simulink model "TV_2021"  (R2017b)
settings: Solver=VariableStepAuto  StartTime=0.0  StopTime=10.0  RelTol=1e-3
undefined symbols (not defined in the file): sigbuilder_block
libraries: simulink x6
(part 6 of 13)

== system TV_2021/Vehicle Dynamics Control 2018/VDC 2018 without Longitudinal/Driver // CarBehaviours ==
  Tq_FRin : Inport
  Tq_FLin : Inport  Port=2
  Tq_RRin : Inport  Port=3
  "Tq_RLin " : Inport  Port=4
  Bp : Inport  Port=5
  Ap : Inport  Port=6
  Reg_enable : Inport  Port=7
  Ap_Sat_up : Inport  Port=8
  Ap_Sat_down : Inport  Port=9
  Accelerating : Subsystem  TreatAsAtomicUnit=on
  "Accelerator behaviour " : MATLAB Function  TreatAsAtomicUnit=on
  Braking Conditions : If  NumInputs=3  IfExpression=u1>0 & u2<0.1 & u3==1  ElseIfExpressions=u1>0 & u2<0.1 & u3==0, u1<0.1 & u2<0.1
  Constant : Constant  Value=0
  Constant1 : Constant  Value=0
  Inertia Braking : Subsystem  TreatAsAtomicUnit=on
  Mech_Braking : Subsystem  TreatAsAtomicUnit=on
  Merge : Merge  Inputs=4
  Merge1 : Merge  Inputs=4
  Regenerative+Mech Braking : Subsystem  TreatAsAtomicUnit=on
  Terminator : Terminator
  Terminator1 : Terminator
  Tq_FRout : Outport
  "Tq_FLout " : Outport  Port=2
  Tq_RRout : Outport  Port=3
  Tq_RLout : Outport  Port=4
  out_Throttle : Outport  Port=5
  wires:
  Constant1/1 -> "Tq_FLout "/1
  Constant/1 -> Tq_FRout/1
  Tq_FLin/1 -> Terminator1/1
  Tq_FRin/1 -> Terminator/1
  Merge/1 -> Tq_RRout/1
  Merge1/1 -> Tq_RLout/1
  Bp/1 -> Braking Conditions/1
  Regenerative+Mech Braking/1("Tq_RR ") -> Merge/1
  Mech_Braking/1("Tq_RR ") -> Merge/2
  Inertia Braking/1("Tq_RR ") -> Merge/3
  Accelerating/1("Tq_RR ") -> Merge/4
  Regenerative+Mech Braking/2(Tq_RL) -> Merge1/1
  Mech_Braking/2(Tq_RL) -> Merge1/2
  Inertia Braking/2(Tq_RL) -> Merge1/3
  Accelerating/2(Tq_RL) -> Merge1/4
  Braking Conditions/1 -> Regenerative+Mech Braking/Action
  Braking Conditions/2 -> Mech_Braking/Action
  Braking Conditions/3 -> Inertia Braking/Action
  Braking Conditions/4 -> Accelerating/Action
  Tq_RRin/1 -> Accelerating/2(Tq_RR), Regenerative+Mech Braking/1(RegTq_RR)
  "Tq_RLin "/1 -> Accelerating/3("Tq_RL "), Regenerative+Mech Braking/2(RegTq_RL)
  Reg_enable/1 -> Braking Conditions/3
  Accelerating/3(Out_Throttle) -> out_Throttle/1
  "Accelerator behaviour "/1(throttle) -> Accelerating/1(Throttle), Braking Conditions/2
  Ap/1 -> "Accelerator behaviour "/1(Ap)
  Ap_Sat_up/1 -> "Accelerator behaviour "/2(Ap_Sat_up)
  Ap_Sat_down/1 -> "Accelerator behaviour "/3(Ap_Sat_down)

== system TV_2021/Vehicle Dynamics Control 2018/VDC 2018 without Longitudinal/In_Numbers ==
  C-Kamm_Factor : Inport
  Max Regen Torque [Nm] : Inport  Port=2
  Limit Power [kW] : Inport  Port=3
  Limit Temperature IGBT [ºC] : Inport  Port=4
  Limit Temperature Motor [ºC] : Inport  Port=5
  Reduction Power [0-1] : Inport  Port=6
  Reduction Temperature [0-1] : Inport  Port=7
  Steering Saturation (per site) [deg] : Inport  Port=8
  Ap_Sat_Down [-] : Inport  Port=9
  Ap_Sat_Up [-] : Inport  Port=10
  3% difference : Gain  Gain=0.97
  Effective Rolling Radius[inch] : Constant  Value=13
  Engine+Inverter Performance [-] : Constant  Value=0.8
  Maximum Torque per engine [Nm] : Constant  Value=140
  Maximum Transmission Torque Dynamic [Nm] : Constant  Value=140
  Maximum Transmission Torque Static [Nm] : Constant  Value=130
  Transmision Ratio[-] : Constant  Value=4
  inch to m : Gain  Gain=0.0254
  Steer_Sat [deg] : Outport
  Tq_Max [Nm] : Outport  Port=2
  Cornering Kamm_Factor [0-2] : Outport  Port=3
  Transmision_Ratio[-] : Outport  Port=4
  Effective Rolling Radius[m] : Outport  Port=5
  Ap_Sat_down[-] : Outport  Port=6
  Ap_Sat_up[-] : Outport  Port=7
  Engine+Inverter Performance[-] : Outport  Port=8
  Trans_max _static[Nm] : Outport  Port=9
  Trans_max_dynamic [Nm] : Outport  Port=10
  "Power limit [KW] " : Outport  Port=11
  Temperature limit IGBT [ºC] : Outport  Port=12
  Temperature limit Motor [ºC] : Outport  Port=13
  Reduction Power (0-1) : Outport  Port=14
  Reduction Temperature (0-1) : Outport  Port=15
  MaxRegTorque [Nm] : Outport  Port=16
  wires:
  Maximum Torque per engine [Nm]/1 -> Tq_Max [Nm]/1
  Transmision Ratio[-]/1 -> Transmision_Ratio[-]/1
  Effective Rolling Radius[inch]/1 -> inch to m/1
  Maximum Transmission Torque Static [Nm]/1 -> Trans_max _static[Nm]/1
  Maximum Transmission Torque Dynamic [Nm]/1 -> Trans_max_dynamic [Nm]/1
  inch to m/1 -> 3% difference/1
  3% difference/1 -> Effective Rolling Radius[m]/1
  Engine+Inverter Performance [-]/1 -> Engine+Inverter Performance[-]/1
  Max Regen Torque [Nm]/1 -> MaxRegTorque [Nm]/1
  Limit Power [kW]/1 -> "Power limit [KW] "/1
  Limit Temperature IGBT [ºC]/1 -> Temperature limit IGBT [ºC]/1
  Reduction Power [0-1]/1 -> Reduction Power (0-1)/1
  C-Kamm_Factor/1 -> Cornering Kamm_Factor [0-2]/1
  Steering Saturation (per site) [deg]/1 -> Steer_Sat [deg]/1
  Ap_Sat_Up [-]/1 -> Ap_Sat_up[-]/1
  Ap_Sat_Down [-]/1 -> Ap_Sat_down[-]/1
  Reduction Temperature [0-1]/1 -> Reduction Temperature (0-1)/1
  Limit Temperature Motor [ºC]/1 -> Temperature limit Motor [ºC]/1

== system TV_2021/Vehicle Dynamics Control 2018/VDC 2018 without Longitudinal/Kamm Circle Lateral ==
  "N_FR " : Inport
  N_FL : Inport  Port=2
  N_RR : Inport  Port=3
  N_RL : Inport  Port=4
  Fy : Inport  Port=5
  CK_Factor : Inport  Port=6
  Constant : Constant  Value=-1
  Constant1 : Constant  Value=-1
  Kamm_Circle LatD : MATLAB Function  TreatAsAtomicUnit=on
  MATLAB Function1 : MATLAB Function  TreatAsAtomicUnit=on
  MATLAB Function2 : MATLAB Function  TreatAsAtomicUnit=on
  Product : Product
  Product1 : Product
  Fx_FR : Outport
  Fx_FL : Outport  Port=2
  "Fx_RR " : Outport  Port=3
  "Fx_RL " : Outport  Port=4
  wires:
  N_FL/1 -> Fx_FL/1
  "N_FR "/1 -> Fx_FR/1
  N_RL/1 -> Kamm_Circle LatD/2(Fz_L)
  Fy/1 -> Kamm_Circle LatD/3(Fy)
  N_RR/1 -> Kamm_Circle LatD/1(Fz_R)
  Kamm_Circle LatD/1(Fx_R) -> Product/1
  Kamm_Circle LatD/2(Fx_L) -> Product1/1
  CK_Factor/1 -> Product/2, Product1/2
  Product1/1 -> MATLAB Function1/2(v)
  Product/1 -> MATLAB Function2/2(v)
  Constant1/1 -> MATLAB Function2/1(cte)
  MATLAB Function2/1(value) -> "Fx_RR "/1
  Constant/1 -> MATLAB Function1/1(cte)
  MATLAB Function1/1(value) -> "Fx_RL "/1

== system TV_2021/Vehicle Dynamics Control 2018/VDC 2018 without Longitudinal/Lateral Dynamics ==
  F_acc : Inport
  R_acc : Inport  Port=2
  FR_susp : Inport  Port=3
  FL_susp : Inport  Port=4
  RR_susp : Inport  Port=5
  RL_susp : Inport  Port=6
  Gas_pedal : Inport  Port=7
  Brake_pedal : Inport  Port=8
  Ellipse_acc : Inport  Port=9
  Constant1 : Constant  Value=0
  Constant2 : Constant  Value=0
  Demux : Demux  Outputs=3
  Demux1 : Demux  Outputs=3
  Fy per wheel : Gain  Gain=1/2
  Gravity : Gain  Gain=1/9.81
  Gravity1 : Gain  Gain=1/9.81
  Product : Product
  Sum : Sum  Inputs=++++
  Sum1 : Sum
  Sum2 : Sum  Inputs=+-
  Terminator{1..7} (7 alike) : Terminator
  N_FR : Outport
  "N_FL " : Outport  Port=2
  "N_RR " : Outport  Port=3
  N_RL : Outport  Port=4
  Fy_R : Outport  Port=5
  Mass [kg] (0,inf) : Outport  Port=6
  Handling [-] (-inf,inf) : Outport  Port=7
  wires:
  Constant2/1 -> "N_FL "/1
  Constant1/1 -> N_FR/1
  F_acc/1 -> Demux1/1
  Gas_pedal/1 -> Terminator4/1
  Brake_pedal/1 -> Terminator5/1
  Demux/2 -> Sum2/2, Product/1
  Demux/1 -> Terminator6/1
  Demux/3 -> Terminator3/1
  Product/1 -> Fy per wheel/1  "Fy per axe"
  Fy per wheel/1 -> Fy_R/1
  Gravity1/1 -> Product/2
  Sum/1 -> Gravity/1
  Sum1/1 -> Gravity1/1
  Gravity/1 -> Mass [kg] (0,inf)/1  "Mass [kg]"
  Demux1/1 -> Terminator1/1
  Demux1/3 -> Terminator2/1
  Demux1/2 -> Sum2/1
  Sum2/1 -> Handling [-] (-inf,inf)/1
  RL_susp/1 -> N_RL/1, Sum1/2, Sum/4
  RR_susp/1 -> Sum1/1, "N_RR "/1, Sum/3
  FL_susp/1 -> Sum/2
  FR_susp/1 -> Sum/1
  R_acc/1 -> Demux/1
  Ellipse_acc/1 -> Terminator7/1

== system TV_2021/Vehicle Dynamics Control 2018/VDC 2018 without Longitudinal/Optimization SKF & CKF ==
  RPM_INV1 : Inport
  RPM_INV2 : Inport  Port=2
  CKF_Initial : Inport  Port=3
  Cte_CKF : Inport  Port=4
  CKF_prev : DataStoreRead  DataStoreName=B
  Data Store Memory1 : DataStoreMemory  DataStoreName=B  ReadBeforeWriteMsg=warning  WriteAfterWriteMsg=warning  WriteAfterReadMsg=warning  ShowAdditionalParam=off
  Data Store Write1 : DataStoreWrite  DataStoreName=B
  Derivative : Derivative
  MATLAB Function : MATLAB Function  TreatAsAtomicUnit=on
  "Subsystem " : Subsystem
  CKF_act : Outport
  wires:
  CKF_prev/1 -> "Subsystem "/3("CKF_prev ")
  Derivative/1 -> "Subsystem "/1(Derivative)  "alpha"
  MATLAB Function/1(RPM) -> Derivative/1  "w (rad/s)"
  "Subsystem "/1(CKF_act) -> Data Store Write1/1, CKF_act/1  "CKF"
  Cte_CKF/1 -> "Subsystem "/4(Cte_CKF)
  CKF_Initial/1 -> "Subsystem "/2("CKF_Initial ")
  RPM_INV1/1 -> MATLAB Function/1(RPM_INV1)
  RPM_INV2/1 -> MATLAB Function/2(RPM_INV2)

== system TV_2021/Vehicle Dynamics Control 2018/VDC 2018 without Longitudinal/Sensor_DATA ==
  note: [ºC]
  note: [m/s2]
  note: [m/s2]
  note: [deg]
  note: [N]
  note: [N]
  note: [N]
  note: [N]
  note: [0-1]
  note: [0-1]
  note: [0 or 1]
  note: [0 - Inf]
  note: [rad/s]
  note: [rad/s]
  Steer_Ang : Inport
  "F_Acc " : Inport  Port=2
  R_Acc : Inport  Port=3
  FR_Susp : Inport  Port=4
  FL_Susp : Inport  Port=5
  RR_Susp : Inport  Port=6
  RL_Susp : Inport  Port=7
  Gas Pedal : Inport  Port=8
  Brake Pedal : Inport  Port=9
  Regenerative Enable : Inport  Port=10
  "Power " : Inport  Port=11
  TemperatureIGBT : Inport  Port=12
  TemperatureMotor : Inport  Port=13
  V_eRR : Inport  Port=14
  "V_eRL " : Inport  Port=15
  Ellipse_acc_ax_ay_az : Inport  Port=16
  Temp_Celdas : Inport  Port=17
  Lim_Temp_Celdas : Inport  Port=18
  Steer_ang : Outport
  F_acc : Outport  Port=2
  R_acc : Outport  Port=3
  FR_susp : Outport  Port=4
  FL_susp : Outport  Port=5
  RR_susp : Outport  Port=6
  RL_susp : Outport  Port=7
  Gas_Pedal : Outport  Port=8
  Brake_Pedal : Outport  Port=9
  Reg_Enable : Outport  Port=10
  Power : Outport  Port=11
  Temperature IGBT : Outport  Port=12
  Temperature Motor : Outport  Port=13
  "V_eRR " : Outport  Port=14
  V_eRL : Outport  Port=15
  Ellipse_acc : Outport  Port=16
  temp_celdas : Outport  Port=17  VectorParamsAs1DForOutWhenUnconnected=on
  Lim_temp_celdas : Outport  Port=18  VectorParamsAs1DForOutWhenUnconnected=on
  wires:
  RL_Susp/1 -> RL_susp/1
  RR_Susp/1 -> RR_susp/1
  FL_Susp/1 -> FL_susp/1
  FR_Susp/1 -> FR_susp/1
  Steer_Ang/1 -> Steer_ang/1
  R_Acc/1 -> R_acc/1
  "F_Acc "/1 -> F_acc/1
  Gas Pedal/1 -> Gas_Pedal/1
  Brake Pedal/1 -> Brake_Pedal/1
  Regenerative Enable/1 -> Reg_Enable/1
  "Power "/1 -> Power/1
  TemperatureIGBT/1 -> Temperature IGBT/1
  "V_eRL "/1 -> V_eRL/1
  V_eRR/1 -> "V_eRR "/1
  TemperatureMotor/1 -> Temperature Motor/1
  Ellipse_acc_ax_ay_az/1 -> Ellipse_acc/1
  Temp_Celdas/1 -> temp_celdas/1
  Lim_Temp_Celdas/1 -> Lim_temp_celdas/1

== system TV_2021/Vehicle Dynamics Control 2018/VDC 2018 without Longitudinal/Wheel_to_engine ==
  "Fx_FR " : Inport
  "Fx_FL " : Inport  Port=2
  "Fx_RR " : Inport  Port=3
  "Fx_RL " : Inport  Port=4
  Re : Inport  Port=5
  RT : Inport  Port=6
  Constant : Constant  Value=0
  Constant1 : Constant  Value=0
  Fx_to_engineTqRL : Subsystem
  Fx_to_engineTqRR : Subsystem
  MATLAB Function1 : MATLAB Function  TreatAsAtomicUnit=on
  MATLAB Function2 : MATLAB Function  TreatAsAtomicUnit=on
  Tq_FR : Outport
  Tq_FL : Outport  Port=2
  Tq_RR : Outport  Port=3
  Tq_RL : Outport  Port=4
  wires:
  Fx_to_engineTqRR/1(Tq) -> Tq_RR/1
  Fx_to_engineTqRL/1(Tq) -> Tq_RL/1
  "Fx_FR "/1 -> Tq_FR/1
  "Fx_FL "/1 -> Tq_FL/1
  Re/1 -> Fx_to_engineTqRR/2(Re), Fx_to_engineTqRL/2(Re)
  RT/1 -> Fx_to_engineTqRR/3(RT), Fx_to_engineTqRL/3(RT)
  "Fx_RR "/1 -> MATLAB Function2/2(v)
  "Fx_RL "/1 -> MATLAB Function1/2(v)
  MATLAB Function2/1(value) -> Fx_to_engineTqRR/1(Fx)
  Constant/1 -> MATLAB Function2/1(cte)
  Constant1/1 -> MATLAB Function1/1(cte)
  MATLAB Function1/1(value) -> Fx_to_engineTqRL/1(Fx)

== system TV_2021/If Action Subsystem1/Steering TV 2017 with TC/Constraints/Control de Potencia  ==
  Tq_RR : Inport
  Tq_RL : Inport  Port=2
  ReductionCte : Inport  Port=3
  Action Port : ActionPort
  Add : Sum  Inputs=+-
  Add1 : Sum  Inputs=+-
  Product : Product
  Product1 : Product
  Tq_RR_out : Outport
  Tq_RL_out : Outport  Port=2
  wires:
  Tq_RR/1 -> Product/1, Add/1
  Tq_RL/1 -> Product1/1, Add1/1
  ReductionCte/1 -> Product/2, Product1/2
  Product1/1 -> Add1/2
  Product/1 -> Add/2
  Add1/1 -> Tq_RL_out/1
  Add/1 -> Tq_RR_out/1

== system TV_2021/If Action Subsystem1/Steering TV 2017 with TC/Constraints/Control de Temperatura ==
  Tq_RR : Inport
  Tq_RL : Inport  Port=2
  ReductionCte : Inport  Port=3
  Action Port : ActionPort
  Add : Sum  Inputs=+-
  Add1 : Sum  Inputs=+-
  Product : Product
  Product1 : Product
  Tq_RR_out : Outport
  Tq_RL_out : Outport  Port=2
  wires:
  Add/1 -> Tq_RR_out/1
  Add1/1 -> Tq_RL_out/1
  Product/1 -> Add/2
  Product1/1 -> Add1/2
  ReductionCte/1 -> Product1/2, Product/2
  Tq_RL/1 -> Add1/1, Product1/1
  Tq_RR/1 -> Add/1, Product/1

== system TV_2021/If Action Subsystem1/Steering TV 2017 with TC/Constraints/else ==
  Tq_RR : Inport
  Tq_RL : Inport  Port=2
  Action Port : ActionPort
  Tq_RR_out : Outport
  Tq_RL_out : Outport  Port=2
  wires:
  Tq_RR/1 -> Tq_RR_out/1
  Tq_RL/1 -> Tq_RL_out/1

== system TV_2021/If Action Subsystem1/Steering TV 2017 with TC/Optimization SKF & CKF/Subsystem  ==
  Steer_An : Inport
  Derivative : Inport  Port=2
  SKF_Initial : Inport  Port=3
  SKF_prev : Inport  Port=4
  "CKF_Initial " : Inport  Port=5
  "CKF_prev " : Inport  Port=6
  Cte_SKF : Inport  Port=7
  Cte_CKF : Inport  Port=8
  CKF : Subsystem
  MATLAB Function1 : MATLAB Function  TreatAsAtomicUnit=on
  SKF : Subsystem
  SKF or CKF : If  IfExpression=-10 < u1 & u1 < 10
  Steering Wheel Maximum Angle : Constant  Value=100
  "SKF_act " : Outport
  CKF_act : Outport  Port=2
  wires:
  MATLAB Function1/1(value) -> SKF or CKF/1
  Steering Wheel Maximum Angle/1 -> MATLAB Function1/1(cte)
  Steer_An/1 -> MATLAB Function1/2(v)
  SKF/1(SKF_act) -> "SKF_act "/1
  CKF/1("CKF_act ") -> CKF_act/1
  SKF or CKF/1 -> SKF/Action
  SKF or CKF/2 -> CKF/Action
  "CKF_prev "/1 -> CKF/3("CKF_prev ")
  Derivative/1 -> CKF/1(Derivative), SKF/1(Derivative)
  SKF_Initial/1 -> SKF/2("SKF_Initial ")
  SKF_prev/1 -> SKF/3(SKF_prev)
  "CKF_Initial "/1 -> CKF/2(CKF_Initial)
  Cte_SKF/1 -> SKF/4(Cte_SKF)
  Cte_CKF/1 -> CKF/4(Cte_CKF)

== system TV_2021/If Action Subsystem1/VDC 2018 Complete/Constraints/Acelerating and braking without Regenerative ==
  Tq_max : Inport
  V_eRR : Inport  Port=2
  V_eRL : Inport  Port=3
  Trans_max_dynamic : Inport  Port=4
  Trans_max_static : Inport  Port=5
  Power_limit : Inport  Port=6
  Power : Inport  Port=7
  Temperature_limit_IGBT : Inport  Port=8
  TemperatureIGBT : Inport  Port=9
  TemperatureI_limit_Motor : Inport  Port=10
  TemperatureMotor : Inport  Port=11
  ReductionCte_Power : Inport  Port=12
  ReductionCte_Temperature : Inport  Port=13
  Tq_FR : Inport  Port=14
  Tq_FL : Inport  Port=15
  Tq_RR : Inport  Port=16
  Tq_RL : Inport  Port=17
  Tq_diff : Inport  Port=18
  Action Port : ActionPort
  "Control de Potencia " : Subsystem  TreatAsAtomicUnit=on
  Control de Temperatura : Subsystem  TreatAsAtomicUnit=on
  Gain : Gain  Gain=3.141592/30
  If : If  NumInputs=6  IfExpression=u4 >= u3 | u6 >= u5  ElseIfExpressions=u2 >= u1
  If Action 1 : Subsystem  TreatAsAtomicUnit=on
  If Action 2 : Subsystem  TreatAsAtomicUnit=on
  If1 : If  NumInputs=3  IfExpression=u1 > u3 & u2 > u3
  Merge{,1,3..4} (4 alike) : Merge  Inputs=3
  Merge2 : Merge
  Momentum Z scaled : Subsystem
  Terminator : Terminator
  Terminator1 : Terminator
  else : Subsystem  TreatAsAtomicUnit=on
  minimum value : MATLAB Function  TreatAsAtomicUnit=on
  minimum value1 : MATLAB Function  TreatAsAtomicUnit=on
  rpm : Constant  Value=200
  TQ_RR : Outport
  TQ_RL : Outport  Port=2
  Flag_Temperature : Outport  Port=3
  Flag_Power : Outport  Port=4
  wires:
  If1/1 -> If Action 1/Action
  If Action 1/1(Trans_limit) -> Merge2/1
  Merge2/1 -> minimum value/1(a), minimum value1/1(a)
  Trans_max_dynamic/1 -> If Action 1/1(Trans_max_dynamic)
  If Action 2/1(Trans_limit) -> Merge2/2
  V_eRR/1 -> If1/1
  V_eRL/1 -> If1/2
  If1/2 -> If Action 2/Action
  Trans_max_static/1 -> If Action 2/1("Trans_max_static ")
  Tq_max/1 -> minimum value1/2(b), minimum value/2(b)
  rpm/1 -> Gain/1
  Gain/1 -> If1/3  "approx 20.95"
  Tq_FR/1 -> Terminator/1
  Tq_FL/1 -> Terminator1/1
  TemperatureIGBT/1 -> If/4
  ReductionCte_Power/1 -> "Control de Potencia "/3(ReductionCte)
  If/3 -> else/Action
  Power_limit/1 -> If/1
  Power/1 -> If/2
  Temperature_limit_IGBT/1 -> If/3
  minimum value/1(min) -> Control de Temperatura/1(Tq_RR), "Control de Potencia "/1(Tq_RR), else/1(Tq_RR)
  minimum value1/1(min) -> Control de Temperatura/2(Tq_RL), "Control de Potencia "/2(Tq_RL), else/2(Tq_RL)
  ReductionCte_Temperature/1 -> Control de Temperatura/3(ReductionCte)
  "Control de Potencia "/1(Tq_RR_out) -> Merge/1
  Control de Temperatura/1(Tq_RR_out) -> Merge/2
  else/1(Tq_RR_out) -> Merge/3
  "Control de Potencia "/2(Tq_RL_out) -> Merge1/1
  Control de Temperatura/2(Tq_RL_out) -> Merge1/2
  else/2(Tq_RL_out) -> Merge1/3
  If/1 -> Control de Temperatura/Action
  If/2 -> "Control de Potencia "/Action
  Tq_RR/1 -> [tq_RR_wc], minimum value/3(c)
  Tq_RL/1 -> [tq_RL_wc], minimum value1/3(c)
  Merge/1 -> Momentum Z scaled/1(Tq_RR_Lim)
  Merge1/1 -> Momentum Z scaled/2(Tq_RL_Lim)
  [tq_RR_wc] -> Momentum Z scaled/3(Tq_RR_wc)
  [tq_RL_wc] -> Momentum Z scaled/4(Tq_RL_wc)
  TemperatureI_limit_Motor/1 -> If/5
  TemperatureMotor/1 -> If/6
  Merge3/1 -> Flag_Temperature/1
  Merge4/1 -> Flag_Power/1
  Control de Temperatura/3(Flag_Temperature) -> Merge3/1
  Control de Temperatura/4(Flag_Power) -> Merge4/1
  "Control de Potencia "/3(Flag_Temperature) -> Merge3/2
  "Control de Potencia "/4(Flag_Power) -> Merge4/2
  else/3(Flag_Temperature) -> Merge3/3
  else/4(Flag_Power) -> Merge4/3
  Momentum Z scaled/1(TQ_RR) -> TQ_RR/1
  Momentum Z scaled/2(TQ_RL) -> TQ_RL/1
  Tq_diff/1 -> Momentum Z scaled/5(Tq_diff)

== system TV_2021/If Action Subsystem1/VDC 2018 Complete/Constraints/Braking with Regenerative ==
  MaxRegTorque : Inport
  Tq_RR_wc : Inport  Port=2
  Tq_RL_wc : Inport  Port=3
  Action Port : ActionPort
  Gain : Gain  Gain=-1
  Gain1 : Gain  Gain=-1
  MATLAB Function : MATLAB Function  TreatAsAtomicUnit=on
  TQ_RR : Outport
  TQ_RL : Outport  Port=2
  wires:
  MATLAB Function/2(RegTq_RL) -> Gain1/1
  MATLAB Function/1(RegTq_RR) -> Gain/1
  Tq_RR_wc/1 -> MATLAB Function/2(Tq_RR)
  Tq_RL_wc/1 -> MATLAB Function/3(Tq_RL)
  MaxRegTorque/1 -> MATLAB Function/1(MaxRegenTq)
  Gain1/1 -> TQ_RL/1
  Gain/1 -> TQ_RR/1

== system TV_2021/If Action Subsystem1/VDC 2018 Complete/Driver // CarBehaviours/Accelerating ==
  Throttle : Inport
  Tq_RR : Inport  Port=2
  "Tq_RL " : Inport  Port=3
  Action Port : ActionPort
  Product : Product
  Product1 : Product
  "Tq_RR " : Outport
  Tq_RL : Outport  Port=2
  Out_Throttle : Outport  Port=3
  wires:
  Product1/1 -> "Tq_RR "/1
  Product/1 -> Tq_RL/1
  Throttle/1 -> Out_Throttle/1, Product/1, Product1/1
  Tq_RR/1 -> Product1/2
  "Tq_RL "/1 -> Product/2

== system TV_2021/If Action Subsystem1/VDC 2018 Complete/Driver // CarBehaviours/Inertia Braking ==
  Action Port : ActionPort
  Constant : Constant  Value=0
  Constant1 : Constant  Value=0
  "Tq_RR " : Outport
  Tq_RL : Outport  Port=2
  wires:
  Constant1/1 -> Tq_RL/1
  Constant/1 -> "Tq_RR "/1

== system TV_2021/If Action Subsystem1/VDC 2018 Complete/Driver // CarBehaviours/Mech_Braking ==
  Action Port : ActionPort
  Constant : Constant  Value=0
  Constant1 : Constant  Value=0
  "Tq_RR " : Outport
  Tq_RL : Outport  Port=2
  wires:
  Constant1/1 -> Tq_RL/1
  Constant/1 -> "Tq_RR "/1

== system TV_2021/If Action Subsystem1/VDC 2018 Complete/Driver // CarBehaviours/Regenerative+Mech Braking ==
  RegTq_RR : Inport
  RegTq_RL : Inport  Port=2
  Action Port : ActionPort
  "Tq_RR " : Outport
  Tq_RL : Outport  Port=2
  wires:
  RegTq_RR/1 -> "Tq_RR "/1
  RegTq_RL/1 -> Tq_RL/1

== system TV_2021/If Action Subsystem1/VDC 2018 Complete/Lateral Dynamics/Kamm_Circle ==
  Fz_R : Inport
  Fz_L : Inport  Port=2
  Fy : Inport  Port=3
  CK_Factor : Inport  Port=4
  Kamm_Circle LatD : MATLAB Function  TreatAsAtomicUnit=on
  Product1 : Product
  Product2 : Product
  Fx_R : Outport
  Fx_L : Outport  Port=2
  Fy_R [N] (0,inf) : Outport  Port=3
  wires:
  Product1/1 -> Fx_R/1
  CK_Factor/1 -> Product1/2, Product2/2
  Product2/1 -> Fx_L/1
  Kamm_Circle LatD/2(Fx_L) -> Product2/1
  Kamm_Circle LatD/1(Fx_R) -> Product1/1
  Fy/1 -> Kamm_Circle LatD/3(Fy)
  Fz_R/1 -> Kamm_Circle LatD/1(Fz_R)
  Fz_L/1 -> Kamm_Circle LatD/2(Fz_L)
  Kamm_Circle LatD/3(Fy_R) -> Fy_R [N] (0,inf)/1

== system TV_2021/If Action Subsystem1/VDC 2018 Complete/Lateral Dynamics/Racecar Model Constants ==
  Wheelbase [m] : Inport
  C. Stiffness [N/rad] : Inport  Port=2
  Steering_Ratio [-] : Inport  Port=3
  L (m) : Outport
  C (N/rad) : Outport  Port=2
  st_ratio (-) : Outport  Port=3
  wires:
  Wheelbase [m]/1 -> L (m)/1
  Steering_Ratio [-]/1 -> st_ratio (-)/1
  C. Stiffness [N/rad]/1 -> C (N/rad)/1

== system TV_2021/If Action Subsystem1/VDC 2018 Complete/Longitudinal Dynamics/Kamm_Circle ==
  Fz_R : Inport
  Fz_L : Inport  Port=2
  Fy : Inport  Port=3
  SK_Factor : Inport  Port=4
  Kamm_Circle LatD : MATLAB Function  TreatAsAtomicUnit=on
  Product : Product
  Product1 : Product
  Fx_R : Outport
  Fx_L : Outport  Port=2
  wires:
  Kamm_Circle LatD/1(Fx_R) -> Product/1
  Kamm_Circle LatD/2(Fx_L) -> Product1/1
  Fz_L/1 -> Kamm_Circle LatD/2(Fz_L)
  Fy/1 -> Kamm_Circle LatD/3(Fy)
  SK_Factor/1 -> Product/2, Product1/2
  Product/1 -> Fx_R/1
  Product1/1 -> Fx_L/1
  Fz_R/1 -> Kamm_Circle LatD/1(Fz_R)

== system TV_2021/If Action Subsystem1/VDC 2018 Complete/Optimization SKF & CKF/Subsystem  ==
  Steer_An : Inport
  Derivative : Inport  Port=2
  SKF_Initial : Inport  Port=3
  SKF_prev : Inport  Port=4
  "CKF_Initial " : Inport  Port=5
  "CKF_prev " : Inport  Port=6
  Cte_SKF : Inport  Port=7
  Cte_CKF : Inport  Port=8
  CKF : Subsystem
  MATLAB Function1 : MATLAB Function  TreatAsAtomicUnit=on
  SKF : Subsystem
  SKF or CKF : If  IfExpression=-10 < u1 & u1 < 10
  Steering Wheel Maximum Angle : Constant  Value=100
  "SKF_act " : Outport
  CKF_act : Outport  Port=2
  wires:
  MATLAB Function1/1(value) -> SKF or CKF/1
  Steering Wheel Maximum Angle/1 -> MATLAB Function1/1(cte)
  Steer_An/1 -> MATLAB Function1/2(v)
  SKF/1(SKF_act) -> "SKF_act "/1
  CKF/1("CKF_act ") -> CKF_act/1
  SKF or CKF/1 -> SKF/Action
  SKF or CKF/2 -> CKF/Action
  "CKF_prev "/1 -> CKF/3("CKF_prev ")
  Derivative/1 -> CKF/1(Derivative), SKF/1(Derivative)
  SKF_Initial/1 -> SKF/2("SKF_Initial ")
  SKF_prev/1 -> SKF/3(SKF_prev)
  "CKF_Initial "/1 -> CKF/2(CKF_Initial)
  Cte_SKF/1 -> SKF/4(Cte_SKF)
  Cte_CKF/1 -> CKF/4(Cte_CKF)

== system TV_2021/If Action Subsystem1/VDC 2018 Complete/Wheel_to_engine/Fx_to_engineTqRL ==
  Fx : Inport
  Re : Inport  Port=2
  RT : Inport  Port=3
  Divide : Product  Inputs=*/
  Product : Product
  Tq : Outport
  wires:
  Divide/1 -> Tq/1
  Product/1 -> Divide/1
  RT/1 -> Divide/2
  Fx/1 -> Product/1
  Re/1 -> Product/2

== system TV_2021/If Action Subsystem1/VDC 2018 Complete/Wheel_to_engine/Fx_to_engineTqRR ==
  Fx : Inport
  Re : Inport  Port=2
  RT : Inport  Port=3
  Divide : Product  Inputs=*/
  Product : Product
  Tq : Outport
  wires:
  Divide/1 -> Tq/1
  Product/1 -> Divide/1
  RT/1 -> Divide/2
  Fx/1 -> Product/1
  Re/1 -> Product/2

== system TV_2021/If Action Subsystem1/VDC 2018 without Longitudinal/Constraints/Acelerating and braking without Regenerative ==
  Tq_max : Inport
  V_eRR : Inport  Port=2
  V_eRL : Inport  Port=3
  Trans_max_dynamic : Inport  Port=4
  Trans_max_static : Inport  Port=5
  Power_limit : Inport  Port=6
  Power : Inport  Port=7
  Temperature_limit_IGBT : Inport  Port=8
  TemperatureIGBT : Inport  Port=9
  TemperatureI_limit_Motor : Inport  Port=10
  TemperatureMotor : Inport  Port=11
  ReductionCte_Power : Inport  Port=12
  ReductionCte_Temperature : Inport  Port=13
  Tq_FR : Inport  Port=14
  Tq_FL : Inport  Port=15
  Tq_RR : Inport  Port=16
  Tq_RL : Inport  Port=17
  Action Port : ActionPort
  "Control de Potencia " : Subsystem  TreatAsAtomicUnit=on
  Control de Temperatura : Subsystem  TreatAsAtomicUnit=on
  Gain : Gain  Gain=3.141592/30
  If : If  NumInputs=6  IfExpression=u4 >= u3 | u6 >= u5  ElseIfExpressions=u2 >= u1
  If Action 1 : Subsystem  TreatAsAtomicUnit=on
  If Action 2 : Subsystem  TreatAsAtomicUnit=on
  If1 : If  NumInputs=3  IfExpression=u1 > u3 & u2 > u3
  Merge : Merge  Inputs=3
  Merge1 : Merge  Inputs=3
  Merge2 : Merge
  Momentum Z scaled : Subsystem
  Terminator : Terminator
  Terminator1 : Terminator
  else : Subsystem  TreatAsAtomicUnit=on
  minimum value : MATLAB Function  TreatAsAtomicUnit=on
  minimum value1 : MATLAB Function  TreatAsAtomicUnit=on
  rpm : Constant  Value=200
  TQ_RR : Outport
  TQ_RL : Outport  Port=2
  wires:
  If1/1 -> If Action 1/Action
  If Action 1/1(Trans_limit) -> Merge2/1
  Merge2/1 -> minimum value/1(a), minimum value1/1(a)
  Trans_max_dynamic/1 -> If Action 1/1(Trans_max_dynamic)
  If Action 2/1(Trans_limit) -> Merge2/2
  V_eRR/1 -> If1/1
  V_eRL/1 -> If1/2
  If1/2 -> If Action 2/Action
  Trans_max_static/1 -> If Action 2/1("Trans_max_static ")
  Tq_max/1 -> minimum value1/2(b), minimum value/2(b)
  rpm/1 -> Gain/1
  Gain/1 -> If1/3  "approx 20.95"
  Tq_FR/1 -> Terminator/1
  Tq_FL/1 -> Terminator1/1
  TemperatureIGBT/1 -> If/4
  ReductionCte_Power/1 -> "Control de Potencia "/3(ReductionCte)
  If/3 -> else/Action
  Power_limit/1 -> If/1
  Power/1 -> If/2
  Temperature_limit_IGBT/1 -> If/3
  minimum value/1(min) -> Control de Temperatura/1(Tq_RR), "Control de Potencia "/1(Tq_RR), else/1(Tq_RR)
  minimum value1/1(min) -> Control de Temperatura/2(Tq_RL), "Control de Potencia "/2(Tq_RL), else/2(Tq_RL)
  ReductionCte_Temperature/1 -> Control de Temperatura/3(ReductionCte)
  "Control de Potencia "/1(Tq_RR_out) -> Merge/1
  Control de Temperatura/1(Tq_RR_out) -> Merge/2
  else/1(Tq_RR_out) -> Merge/3
  "Control de Potencia "/2(Tq_RL_out) -> Merge1/1
  Control de Temperatura/2(Tq_RL_out) -> Merge1/2
  else/2(Tq_RL_out) -> Merge1/3
  If/1 -> Control de Temperatura/Action
  If/2 -> "Control de Potencia "/Action
  Tq_RR/1 -> [tq_RR_wc], minimum value/3(c)
  Tq_RL/1 -> [tq_RL_wc], minimum value1/3(c)
  Merge/1 -> Momentum Z scaled/1(Tq_RR_Lim)
  Merge1/1 -> Momentum Z scaled/2(Tq_RL_Lim)
  [tq_RR_wc] -> Momentum Z scaled/3(Tq_RR_wc)
  [tq_RL_wc] -> Momentum Z scaled/4(Tq_RL_wc)
  TemperatureI_limit_Motor/1 -> If/5
  TemperatureMotor/1 -> If/6
  Momentum Z scaled/1(TQ_RR) -> TQ_RR/1
  Momentum Z scaled/2(TQ_RL) -> TQ_RL/1

== system TV_2021/If Action Subsystem1/VDC 2018 without Longitudinal/Constraints/Braking with Regenerative ==
  MaxRegTorque : Inport
  Tq_RR_wc : Inport  Port=2
  Tq_RL_wc : Inport  Port=3
  Action Port : ActionPort
  Gain : Gain  Gain=-1
  Gain1 : Gain  Gain=-1
  MATLAB Function : MATLAB Function  TreatAsAtomicUnit=on
  TQ_RR : Outport
  TQ_RL : Outport  Port=2
  wires:
  MATLAB Function/2(RegTq_RL) -> Gain1/1
  MATLAB Function/1(RegTq_RR) -> Gain/1
  Tq_RR_wc/1 -> MATLAB Function/2(Tq_RR)
  Tq_RL_wc/1 -> MATLAB Function/3(Tq_RL)
  MaxRegTorque/1 -> MATLAB Function/1(MaxRegenTq)
  Gain1/1 -> TQ_RL/1
  Gain/1 -> TQ_RR/1

== system TV_2021/If Action Subsystem1/VDC 2018 without Longitudinal/Driver // CarBehaviours/Accelerating ==
  Ap : Inport
  "Ap_Sat_up " : Inport  Port=2
  Ap_Sat_down : Inport  Port=3
  Tq_RR : Inport  Port=4
  "Tq_RL " : Inport  Port=5
  Action Port : ActionPort
  "Accelerator behaviour " : MATLAB Function  TreatAsAtomicUnit=on
  Product : Product
  Product1 : Product
  "Tq_RR " : Outport
  Tq_RL : Outport  Port=2
  Out_Throttle : Outport  Port=3
  wires:
  Ap/1 -> "Accelerator behaviour "/1(Ap)
  "Ap_Sat_up "/1 -> "Accelerator behaviour "/2(Ap_Sat_up)
  Ap_Sat_down/1 -> "Accelerator behaviour "/3(Ap_Sat_down)
  Product1/1 -> "Tq_RR "/1
  Product/1 -> Tq_RL/1
  "Accelerator behaviour "/1(throttle) -> Out_Throttle/1, Product/1, Product1/1
  Tq_RR/1 -> Product1/2
  "Tq_RL "/1 -> Product/2

== system TV_2021/If Action Subsystem1/VDC 2018 without Longitudinal/Driver // CarBehaviours/Inertia Braking ==
  Action Port : ActionPort
  Constant : Constant  Value=0
  Constant1 : Constant  Value=0
  "Tq_RR " : Outport
  Tq_RL : Outport  Port=2
  wires:
  Constant1/1 -> Tq_RL/1
  Constant/1 -> "Tq_RR "/1

== system TV_2021/If Action Subsystem1/VDC 2018 without Longitudinal/Driver // CarBehaviours/Mech_Braking ==
  Action Port : ActionPort
  Constant : Constant  Value=0
  Constant1 : Constant  Value=0
  "Tq_RR " : Outport
  Tq_RL : Outport  Port=2
  wires:
  Constant1/1 -> Tq_RL/1
  Constant/1 -> "Tq_RR "/1

== system TV_2021/If Action Subsystem1/VDC 2018 without Longitudinal/Driver // CarBehaviours/Regenerative+Mech Braking ==
  RegTq_RR : Inport
  RegTq_RL : Inport  Port=2
  Action Port : ActionPort
  "Tq_RR " : Outport
  Tq_RL : Outport  Port=2
  wires:
  RegTq_RL/1 -> Tq_RL/1
  RegTq_RR/1 -> "Tq_RR "/1

== system TV_2021/If Action Subsystem1/VDC 2018 without Longitudinal/Optimization SKF & CKF/Subsystem  ==
  Derivative : Inport
  "CKF_Initial " : Inport  Port=2
  "CKF_prev " : Inport  Port=3
  Cte_CKF : Inport  Port=4
  CKF : Subsystem
  CKF_act : Outport
  wires:
  CKF/1("CKF_act ") -> CKF_act/1
  "CKF_prev "/1 -> CKF/3("CKF_prev ")
  Derivative/1 -> CKF/1(Derivative)
  "CKF_Initial "/1 -> CKF/2(CKF_Initial)
  Cte_CKF/1 -> CKF/4(Cte_CKF)

== system TV_2021/If Action Subsystem1/VDC 2018 without Longitudinal/Wheel_to_engine/Fx_to_engineTqRL ==
  Fx : Inport
  Re : Inport  Port=2
  RT : Inport  Port=3
  Divide : Product  Inputs=*/
  Product : Product
  Tq : Outport
  wires:
  Divide/1 -> Tq/1
  Product/1 -> Divide/1
  RT/1 -> Divide/2
  Fx/1 -> Product/1
  Re/1 -> Product/2

== system TV_2021/If Action Subsystem1/VDC 2018 without Longitudinal/Wheel_to_engine/Fx_to_engineTqRR ==
  Fx : Inport
  Re : Inport  Port=2
  RT : Inport  Port=3
  Divide : Product  Inputs=*/
  Product : Product
  Tq : Outport
  wires:
  Divide/1 -> Tq/1
  Product/1 -> Divide/1
  RT/1 -> Divide/2
  Fx/1 -> Product/1
  Re/1 -> Product/2

== system TV_2021/Vehicle Dynamics Control 1/Steering TV 2017 with TC/Constraints/Control de Potencia  ==
  Tq_RR : Inport
  Tq_RL : Inport  Port=2
  ReductionCte : Inport  Port=3
  Action Port : ActionPort
  Add : Sum  Inputs=+-
  Add1 : Sum  Inputs=+-
  Product : Product
  Product1 : Product
  Tq_RR_out : Outport
  Tq_RL_out : Outport  Port=2
  wires:
  Add/1 -> Tq_RR_out/1
  Add1/1 -> Tq_RL_out/1
  Product/1 -> Add/2
  Product1/1 -> Add1/2
  ReductionCte/1 -> Product1/2, Product/2
  Tq_RL/1 -> Add1/1, Product1/1
  Tq_RR/1 -> Add/1, Product/1

== system TV_2021/Vehicle Dynamics Control 1/Steering TV 2017 with TC/Constraints/Control de Temperatura ==
  Tq_RR : Inport
  Tq_RL : Inport  Port=2
  ReductionCte : Inport  Port=3
  Action Port : ActionPort
  Add : Sum  Inputs=+-
  Add1 : Sum  Inputs=+-
  Product : Product
  Product1 : Product
  Tq_RR_out : Outport
  Tq_RL_out : Outport  Port=2
  wires:
  Add/1 -> Tq_RR_out/1
  ReductionCte/1 -> Product/2, Product1/2
  Tq_RL/1 -> Product1/1, Add1/1
  Tq_RR/1 -> Product/1, Add/1
  Add1/1 -> Tq_RL_out/1
  Product1/1 -> Add1/2
  Product/1 -> Add/2

== system TV_2021/Vehicle Dynamics Control 1/Steering TV 2017 with TC/Constraints/current_limitation1 ==
  note: % de la corriente total que te dejo usar
  max_cell_temp : Inport
  actual_current : Inport  Port=2
  initial_limitation : Inport  Port=3
  max_discharge_current : Inport  Port=4
  max_regen_current : Inport  Port=5
  Product1 : Product
  constants_saturator : Subsystem
  temperature_rise_limitator : Subsystem
  max_discharge (-) : Outport  VectorParamsAs1DForOutWhenUnconnected=on
  max_regen (+) : Outport  Port=2  VectorParamsAs1DForOutWhenUnconnected=on
  fans_control : Outport  Port=3  VectorParamsAs1DForOutWhenUnconnected=on
  wires:
  temperature_rise_limitator/1(allowed_current) -> Product1/1, fans_control/1
  max_regen_current/1 -> constants_saturator/3(max_regen_current)
  max_discharge_current/1 -> constants_saturator/2(max_discharge_current)
  initial_limitation/1 -> temperature_rise_limitator/2(initial_limitation)
  constants_saturator/2(limited_regen_actual) -> max_regen (+)/1
  constants_saturator/1(limited_discharge_actual) -> max_discharge (-)/1
  Product1/1 -> constants_saturator/1(allowed_current [%])
  max_cell_temp/1 -> temperature_rise_limitator/1(max_cell_temp)
  actual_current/1 -> Product1/2

== system TV_2021/Vehicle Dynamics Control 1/Steering TV 2017 with TC/Constraints/else ==
  Tq_RR : Inport
  Tq_RL : Inport  Port=2
  Action Port : ActionPort
  Tq_RR_out : Outport
  Tq_RL_out : Outport  Port=2
  wires:
  Tq_RL/1 -> Tq_RL_out/1
  Tq_RR/1 -> Tq_RR_out/1

== system TV_2021/Vehicle Dynamics Control 1/Steering TV 2017 with TC/Optimization SKF & CKF/Subsystem  ==
  Steer_An : Inport
  Derivative : Inport  Port=2
  SKF_Initial : Inport  Port=3
  SKF_prev : Inport  Port=4
  "CKF_Initial " : Inport  Port=5
  "CKF_prev " : Inport  Port=6
  Cte_SKF : Inport  Port=7
  Cte_CKF : Inport  Port=8
  CKF : Subsystem
  MATLAB Function1 : MATLAB Function  TreatAsAtomicUnit=on
  SKF : Subsystem
  SKF or CKF : If  IfExpression=-10 < u1 & u1 < 10
  Steering Wheel Maximum Angle : Constant  Value=100
  "SKF_act " : Outport
  CKF_act : Outport  Port=2
  wires:
  Cte_CKF/1 -> CKF/4(Cte_CKF)
  Cte_SKF/1 -> SKF/4(Cte_SKF)
  "CKF_Initial "/1 -> CKF/2(CKF_Initial)
  SKF_prev/1 -> SKF/3(SKF_prev)
  SKF_Initial/1 -> SKF/2("SKF_Initial ")
  Derivative/1 -> SKF/1(Derivative), CKF/1(Derivative)
  "CKF_prev "/1 -> CKF/3("CKF_prev ")
  SKF or CKF/2 -> CKF/Action
  SKF or CKF/1 -> SKF/Action
  CKF/1("CKF_act ") -> CKF_act/1
  SKF/1(SKF_act) -> "SKF_act "/1
  Steer_An/1 -> MATLAB Function1/2(v)
  Steering Wheel Maximum Angle/1 -> MATLAB Function1/1(cte)
  MATLAB Function1/1(value) -> SKF or CKF/1

== system TV_2021/Vehicle Dynamics Control 1/VDC 2018 Complete/Constraints/Acelerating and braking without Regenerative ==
  Tq_max : Inport
  V_eRR : Inport  Port=2
  V_eRL : Inport  Port=3
  Trans_max_dynamic : Inport  Port=4
  Trans_max_static : Inport  Port=5
  Power_limit : Inport  Port=6
  Power : Inport  Port=7
  Temperature_limit_IGBT : Inport  Port=8
  TemperatureIGBT : Inport  Port=9
  TemperatureI_limit_Motor : Inport  Port=10
  TemperatureMotor : Inport  Port=11
  ReductionCte_Power : Inport  Port=12
  ReductionCte_Temperature : Inport  Port=13
  Tq_FR : Inport  Port=14
  Tq_FL : Inport  Port=15
  Tq_RR : Inport  Port=16
  Tq_RL : Inport  Port=17
  Tq_diff : Inport  Port=18
  Tq_diff_max : Inport  Port=19
  Temp_celdas : Inport  Port=20
  Limit_Temp_celdas : Inport  Port=21
  Action Port : ActionPort
  "Control de Potencia " : Subsystem  TreatAsAtomicUnit=on
  Control de Temperatura : Subsystem  TreatAsAtomicUnit=on
  Gain : Gain  Gain=3.141592/30
  If : If  NumInputs=8  IfExpression=u4 >= u3 | u6 >= u5 | u7>=u8  ElseIfExpressions=u2 >= u1
  If Action 1 : Subsystem  TreatAsAtomicUnit=on
  If Action 2 : Subsystem  TreatAsAtomicUnit=on
  If1 : If  NumInputs=3  IfExpression=u1 > u3 & u2 > u3
  MATLAB Function : MATLAB Function  TreatAsAtomicUnit=on
  Merge{,1,3..4} (4 alike) : Merge  Inputs=3
  Merge2 : Merge
  Momentum Z scaled : Subsystem
  Terminator : Terminator
  Terminator1 : Terminator
  else : Subsystem  TreatAsAtomicUnit=on
  minimum value : MATLAB Function  TreatAsAtomicUnit=on
  minimum value1 : MATLAB Function  TreatAsAtomicUnit=on
  rpm : Constant  Value=200
  TQ_RR : Outport
  TQ_RL : Outport  Port=2
  Flag_Temperature : Outport  Port=3
  Flag_Power : Outport  Port=4
  wires:
  Limit_Temp_celdas/1 -> If/8
  Temp_celdas/1 -> If/7
  [Tq_diff_lim] -> Momentum Z scaled/5(Tq_diff)
  MATLAB Function/1(diff_lim) -> [Tq_diff_lim]
  Tq_diff_max/1 -> MATLAB Function/2(diff_max)
  Tq_diff/1 -> MATLAB Function/1(diff_wc)
  Momentum Z scaled/2(TQ_RL) -> TQ_RL/1
  Momentum Z scaled/1(TQ_RR) -> TQ_RR/1
  else/4(Flag_Power) -> Merge4/3
  else/3(Flag_Temperature) -> Merge3/3
  "Control de Potencia "/4(Flag_Power) -> Merge4/2
  "Control de Potencia "/3(Flag_Temperature) -> Merge3/2
  Control de Temperatura/4(Flag_Power) -> Merge4/1
  Control de Temperatura/3(Flag_Temperature) -> Merge3/1
  Merge4/1 -> Flag_Power/1
  Merge3/1 -> Flag_Temperature/1
  TemperatureMotor/1 -> If/6
  TemperatureI_limit_Motor/1 -> If/5
  [tq_RL_wc] -> Momentum Z scaled/4(Tq_RL_wc)
  [tq_RR_wc] -> Momentum Z scaled/3(Tq_RR_wc)
  Merge1/1 -> Momentum Z scaled/2(Tq_RL_Lim)
  Merge/1 -> Momentum Z scaled/1(Tq_RR_Lim)
  Tq_RL/1 -> minimum value1/3(c), [tq_RL_wc]
  Tq_RR/1 -> minimum value/3(c), [tq_RR_wc]
  If/2 -> "Control de Potencia "/Action
  If/1 -> Control de Temperatura/Action
  else/2(Tq_RL_out) -> Merge1/3
  Control de Temperatura/2(Tq_RL_out) -> Merge1/2
  "Control de Potencia "/2(Tq_RL_out) -> Merge1/1
  else/1(Tq_RR_out) -> Merge/3
  Control de Temperatura/1(Tq_RR_out) -> Merge/2
  "Control de Potencia "/1(Tq_RR_out) -> Merge/1
  ReductionCte_Temperature/1 -> Control de Temperatura/3(ReductionCte)
  minimum value1/1(min) -> else/2(Tq_RL), "Control de Potencia "/2(Tq_RL), Control de Temperatura/2(Tq_RL)
  minimum value/1(min) -> else/1(Tq_RR), "Control de Potencia "/1(Tq_RR), Control de Temperatura/1(Tq_RR)
  Temperature_limit_IGBT/1 -> If/3
  Power/1 -> If/2
  Power_limit/1 -> If/1
  If/3 -> else/Action
  ReductionCte_Power/1 -> "Control de Potencia "/3(ReductionCte)
  TemperatureIGBT/1 -> If/4
  Tq_FL/1 -> Terminator1/1
  Tq_FR/1 -> Terminator/1
  Gain/1 -> If1/3  "approx 20.95"
  rpm/1 -> Gain/1
  Tq_max/1 -> minimum value/2(b), minimum value1/2(b)
  Trans_max_static/1 -> If Action 2/1("Trans_max_static ")
  If1/2 -> If Action 2/Action
  V_eRL/1 -> If1/2
  V_eRR/1 -> If1/1
  If Action 2/1(Trans_limit) -> Merge2/2
  Trans_max_dynamic/1 -> If Action 1/1(Trans_max_dynamic)
  Merge2/1 -> minimum value1/1(a), minimum value/1(a)
  If Action 1/1(Trans_limit) -> Merge2/1
  If1/1 -> If Action 1/Action

== system TV_2021/Vehicle Dynamics Control 1/VDC 2018 Complete/Constraints/Braking with Regenerative ==
  MaxRegTorque : Inport
  Tq_RR_wc : Inport  Port=2
  Tq_RL_wc : Inport  Port=3
  Action Port : ActionPort
  Gain : Gain  Gain=-1
  Gain1 : Gain  Gain=-1
  MATLAB Function : MATLAB Function  TreatAsAtomicUnit=on
  TQ_RR : Outport
  TQ_RL : Outport  Port=2
  wires:
  Gain/1 -> TQ_RR/1
  Gain1/1 -> TQ_RL/1
  MaxRegTorque/1 -> MATLAB Function/1(MaxRegenTq)
  Tq_RL_wc/1 -> MATLAB Function/3(Tq_RL)
  Tq_RR_wc/1 -> MATLAB Function/2(Tq_RR)
  MATLAB Function/1(RegTq_RR) -> Gain/1
  MATLAB Function/2(RegTq_RL) -> Gain1/1

== system TV_2021/Vehicle Dynamics Control 1/VDC 2018 Complete/Driver // CarBehaviours/Accelerating ==
  Throttle : Inport
  Tq_RR : Inport  Port=2
  "Tq_RL " : Inport  Port=3
  Action Port : ActionPort
  Product : Product
  Product1 : Product
  "Tq_RR " : Outport
  Tq_RL : Outport  Port=2
  Out_Throttle : Outport  Port=3
  wires:
  "Tq_RL "/1 -> Product/2
  Tq_RR/1 -> Product1/2
  Throttle/1 -> Product1/1, Product/1, Out_Throttle/1
  Product/1 -> Tq_RL/1
  Product1/1 -> "Tq_RR "/1

== system TV_2021/Vehicle Dynamics Control 1/VDC 2018 Complete/Driver // CarBehaviours/Inertia Braking ==
  Action Port : ActionPort
  Constant : Constant  Value=0
  Constant1 : Constant  Value=0
  "Tq_RR " : Outport
  Tq_RL : Outport  Port=2
  wires:
  Constant/1 -> "Tq_RR "/1
  Constant1/1 -> Tq_RL/1

== system TV_2021/Vehicle Dynamics Control 1/VDC 2018 Complete/Driver // CarBehaviours/Mech_Braking ==
  Action Port : ActionPort
  Constant : Constant  Value=0
  Constant1 : Constant  Value=0
  "Tq_RR " : Outport
  Tq_RL : Outport  Port=2
  wires:
  Constant/1 -> "Tq_RR "/1
  Constant1/1 -> Tq_RL/1

== system TV_2021/Vehicle Dynamics Control 1/VDC 2018 Complete/Driver // CarBehaviours/Regenerative+Mech Braking ==
  RegTq_RR : Inport
  RegTq_RL : Inport  Port=2
  Action Port : ActionPort
  "Tq_RR " : Outport
  Tq_RL : Outport  Port=2
  wires:
  RegTq_RL/1 -> Tq_RL/1
  RegTq_RR/1 -> "Tq_RR "/1

== system TV_2021/Vehicle Dynamics Control 1/VDC 2018 Complete/Lateral Dynamics/Kamm_Circle ==
  Fz_R : Inport
  Fz_L : Inport  Port=2
  Fy : Inport  Port=3
  CK_Factor : Inport  Port=4
  Kamm_Circle LatD : MATLAB Function  TreatAsAtomicUnit=on
  Product1 : Product
  Product2 : Product
  Fx_R : Outport
  Fx_L : Outport  Port=2
  Fy_R [N] (0,inf) : Outport  Port=3
  wires:
  Product1/1 -> Fx_R/1
  CK_Factor/1 -> Product1/2, Product2/2
  Product2/1 -> Fx_L/1
  Kamm_Circle LatD/2(Fx_L) -> Product2/1
  Kamm_Circle LatD/1(Fx_R) -> Product1/1
  Fy/1 -> Kamm_Circle LatD/3(Fy)
  Fz_R/1 -> Kamm_Circle LatD/1(Fz_R)
  Fz_L/1 -> Kamm_Circle LatD/2(Fz_L)
  Kamm_Circle LatD/3(Fy_R) -> Fy_R [N] (0,inf)/1

== system TV_2021/Vehicle Dynamics Control 1/VDC 2018 Complete/Lateral Dynamics/Tire Longitudinal Force Difference ==
  e : Inport
  Iz : Inport  Port=2
  dt : Inport  Port=3
  rt : Inport  Port=4
  " Momentum_Z to Longitudinal Force Difference" : Subsystem
  Momentum respect to Z-axis to correct the error : Subsystem
  Scope5 : Scope
  Scope6 : Scope
  Fx_diff : Outport
  wires:
  e/1 -> Momentum respect to Z-axis to correct the error/1(Yaw_error_[º/s]), Scope5/1
  Momentum respect to Z-axis to correct the error/1(Momentum_Z [Nm]) -> Scope6/1, " Momentum_Z to Longitudinal Force Difference"/1("\tMomentumZ [Nm]")
  Iz/1 -> Momentum respect to Z-axis to correct the error/2(Iz [kg/m^3])
  " Momentum_Z to Longitudinal Force Difference"/1(Fx_diff [N]) -> Fx_diff/1
  rt/1 -> " Momentum_Z to Longitudinal Force Difference"/2(RearTrackwidth [m])
  dt/1 -> Momentum respect to Z-axis to correct the error/3(Correction_Time [s])

== system TV_2021/Vehicle Dynamics Control 1/VDC 2018 Complete/Lateral Dynamics/Yaw_Rate_Reference ==
  Steering_Angle : Inport
  F_vel_x : Inport  Port=2
  360/(2*pi) : Gain  Gain=360/(2*pi)
  360/(2pi) : Gain  Gain=360/(2*pi)
  Bicycle Model : MATLAB Function  TreatAsAtomicUnit=on
  Constant7 : Constant  Value=0.92
  Constant8 : Constant  Value=360
  Cornering_Stiffness_F[N/º] : Constant  Value=-700
  Cornering_Stiffness_R[N/º] : Constant  Value=-1000
  Divide : Product  Inputs=*/
  Gain{,1..4} (5 alike) : Gain  Gain=360/(2*pi)
  Scope1 : Scope  NumInputPorts=5
  Scope2 : Scope  NumInputPorts=2
  Scope3 : Scope
  Steering_Ratio [-] : Constant  Value=3.72
  Wheelbase [m] : Constant  Value=1.53
  Yaw_Rate : Outport
  wires:
  Bicycle Model/8(yr) -> Scope2/2
  Steering_Angle/1 -> Divide/1
  Wheelbase [m]/1 -> Bicycle Model/5(L)
  Divide/1 -> Bicycle Model/1(delta), Gain1/1
  Bicycle Model/1(r) -> Yaw_Rate/1
  Steering_Ratio [-]/1 -> Divide/2
  Bicycle Model/4(alpha_r) -> Gain3/1
  Constant8/1 -> Bicycle Model/3(m)
  Bicycle Model/5(course) -> Gain/1
  Constant7/1 -> Bicycle Model/4(xCG)
  Cornering_Stiffness_F[N/º]/1 -> 360/(2*pi)/1
  Bicycle Model/6(radius) -> Scope3/1
  Bicycle Model/3(alpha_f) -> Gain4/1
  Bicycle Model/7(yf) -> Scope2/1
  F_vel_x/1 -> Bicycle Model/2(vx)
  Bicycle Model/2(beta) -> Gain2/1
  360/(2*pi)/1 -> Bicycle Model/6(cf)
  Cornering_Stiffness_R[N/º]/1 -> 360/(2pi)/1
  360/(2pi)/1 -> Bicycle Model/7(cr)
  Gain/1 -> Scope1/5
  Gain1/1 -> Scope1/1
  Gain2/1 -> Scope1/4
  Gain3/1 -> Scope1/3
  Gain4/1 -> Scope1/2

== system TV_2021/Vehicle Dynamics Control 1/VDC 2018 Complete/Longitudinal Dynamics/Kamm_Circle ==
  Fz_R : Inport
  Fz_L : Inport  Port=2
  Fy : Inport  Port=3
  SK_Factor : Inport  Port=4
  Kamm_Circle LatD : MATLAB Function  TreatAsAtomicUnit=on
  Product : Product
  Product1 : Product
  Fx_R : Outport
  Fx_L : Outport  Port=2
  wires:
  Fz_R/1 -> Kamm_Circle LatD/1(Fz_R)
  Product1/1 -> Fx_L/1
  Product/1 -> Fx_R/1
  SK_Factor/1 -> Product1/2, Product/2
  Fy/1 -> Kamm_Circle LatD/3(Fy)
  Fz_L/1 -> Kamm_Circle LatD/2(Fz_L)
  Kamm_Circle LatD/2(Fx_L) -> Product1/1
  Kamm_Circle LatD/1(Fx_R) -> Product/1

== system TV_2021/Vehicle Dynamics Control 1/VDC 2018 Complete/Optimization SKF & CKF/Subsystem  ==
  Steer_An : Inport
  Derivative : Inport  Port=2
  SKF_Initial : Inport  Port=3
  SKF_prev : Inport  Port=4
  "CKF_Initial " : Inport  Port=5
  "CKF_prev " : Inport  Port=6
  Cte_SKF : Inport  Port=7
  Cte_CKF : Inport  Port=8
  CKF : Subsystem
  MATLAB Function1 : MATLAB Function  TreatAsAtomicUnit=on
  SKF : Subsystem
  SKF or CKF : If  IfExpression=-10 < u1 & u1 < 10
  Steering Wheel Maximum Angle : Constant  Value=100
  "SKF_act " : Outport
  CKF_act : Outport  Port=2
  wires:
  Cte_CKF/1 -> CKF/4(Cte_CKF)
  Cte_SKF/1 -> SKF/4(Cte_SKF)
  "CKF_Initial "/1 -> CKF/2(CKF_Initial)
  SKF_prev/1 -> SKF/3(SKF_prev)
  SKF_Initial/1 -> SKF/2("SKF_Initial ")
  Derivative/1 -> SKF/1(Derivative), CKF/1(Derivative)
  "CKF_prev "/1 -> CKF/3("CKF_prev ")
  SKF or CKF/2 -> CKF/Action
  SKF or CKF/1 -> SKF/Action
  CKF/1("CKF_act ") -> CKF_act/1
  SKF/1(SKF_act) -> "SKF_act "/1
  Steer_An/1 -> MATLAB Function1/2(v)
  Steering Wheel Maximum Angle/1 -> MATLAB Function1/1(cte)
  MATLAB Function1/1(value) -> SKF or CKF/1

== system TV_2021/Vehicle Dynamics Control 1/VDC 2018 Complete/Wheel_to_engine/Fx_to_engineTqRL ==
  Fx : Inport
  Re : Inport  Port=2
  RT : Inport  Port=3
  Divide : Product  Inputs=*/
  Product : Product
  Tq : Outport
  wires:
  Re/1 -> Product/2
  Fx/1 -> Product/1
  RT/1 -> Divide/2
  Product/1 -> Divide/1
  Divide/1 -> Tq/1

== system TV_2021/Vehicle Dynamics Control 1/VDC 2018 Complete/Wheel_to_engine/Fx_to_engineTqRR ==
  Fx : Inport
  Re : Inport  Port=2
  RT : Inport  Port=3
  Divide : Product  Inputs=*/
  Product : Product
  Tq : Outport
  wires:
  Re/1 -> Product/2
  Fx/1 -> Product/1
  RT/1 -> Divide/2
  Product/1 -> Divide/1
  Divide/1 -> Tq/1

== system TV_2021/Vehicle Dynamics Control 1/VDC 2018 without Longitudinal/Constraints/Acelerating and braking without Regenerative ==
  note: Considero de la misma gravedad,
      | la limitacion por potencia que por temperatura
  Tq_max : Inport
  V_eRR : Inport  Port=2
  V_eRL : Inport  Port=3
  Trans_max_dynamic : Inport  Port=4
  Trans_max_static : Inport  Port=5
  Tq_FR : Inport  Port=6
  Tq_FL : Inport  Port=7
  Tq_RR : Inport  Port=8
  Tq_RL : Inport  Port=9
  Power_limit1 : Inport  Port=10
  Power1 : Inport  Port=11
  Temperature_limit_IGBT1 : Inport  Port=12
  Temperature_IGBT : Inport  Port=13
  Temperature_limit_Motor : Inport  Port=14
  Temperature_Motor : Inport  Port=15
  Temp_Celdas : Inport  Port=16
  Lim_Temp_Celdas : Inport  Port=17
  ReductionCte_Temperature1 : Inport  Port=18
  ReductionCte_Power1 : Inport  Port=19
  Action Port : ActionPort
  Control de Potencia 1 : Subsystem  TreatAsAtomicUnit=on
  Control de Temperatura1 : Subsystem  TreatAsAtomicUnit=on
  Gain : Gain  Gain=3.141592/30
  If Action 1 : Subsystem  TreatAsAtomicUnit=on
  If Action 2 : Subsystem  TreatAsAtomicUnit=on
  If1 : If  NumInputs=3  IfExpression=u1 > u3 & u2 > u3
  If2 : If  NumInputs=8  IfExpression=u4 >= u3 | u6 >= u5 | u7>=u8  ElseIfExpressions=u2 >= u1
  Merge2 : Merge
  Merge3 : Merge  Inputs=3
  Merge4 : Merge  Inputs=3
  Momentum Z scaled : Subsystem
  Terminator : Terminator
  Terminator1 : Terminator
  else1 : Subsystem  TreatAsAtomicUnit=on
  minimum value : MATLAB Function  TreatAsAtomicUnit=on
  minimum value1 : MATLAB Function  TreatAsAtomicUnit=on
  rpm : Constant  Value=200
  TQ_RR : Outport
  TQ_RL : Outport  Port=2
  wires:
  Power_limit1/1 -> If2/1
  Control de Potencia 1/2(Tq_RL_out) -> Merge4/1
  Temperature_IGBT/1 -> If2/4
  minimum value1/1(min) -> else1/2(Tq_RL), Control de Potencia 1/2(Tq_RL), Control de Temperatura1/2(Tq_RL)
  ReductionCte_Power1/1 -> Control de Potencia 1/3(ReductionCte)
  Power1/1 -> If2/2
  Temperature_limit_IGBT1/1 -> If2/3
  If2/1 -> Control de Temperatura1/Action
  ReductionCte_Temperature1/1 -> Control de Temperatura1/3(ReductionCte)
  Control de Potencia 1/1(Tq_RR_out) -> Merge3/1
  minimum value/1(min) -> else1/1(Tq_RR), Control de Potencia 1/1(Tq_RR), Control de Temperatura1/1(Tq_RR)
  else1/2(Tq_RL_out) -> Merge4/3
  If2/3 -> else1/Action
  If2/2 -> Control de Potencia 1/Action
  Control de Temperatura1/2(Tq_RL_out) -> Merge4/2
  else1/1(Tq_RR_out) -> Merge3/3
  Temperature_Motor/1 -> If2/6
  Temperature_limit_Motor/1 -> If2/5
  Control de Temperatura1/1(Tq_RR_out) -> Merge3/2
  Lim_Temp_Celdas/1 -> If2/8
  Temp_Celdas/1 -> If2/7
  Momentum Z scaled/2(TQ_RL) -> TQ_RL/1
  Momentum Z scaled/1(TQ_RR) -> TQ_RR/1
  [tq_RL_wc] -> Momentum Z scaled/4(Tq_RL_wc)
  [tq_RR_wc] -> Momentum Z scaled/3(Tq_RR_wc)
  Merge4/1 -> Momentum Z scaled/2(Tq_RL_Lim)
  Merge3/1 -> Momentum Z scaled/1(Tq_RR_Lim)
  Tq_RL/1 -> minimum value1/3(c), [tq_RL_wc]
  Tq_RR/1 -> minimum value/3(c), [tq_RR_wc]
  Tq_FL/1 -> Terminator1/1
  Tq_FR/1 -> Terminator/1
  Gain/1 -> If1/3  "approx 20.95"
  rpm/1 -> Gain/1
  Tq_max/1 -> minimum value/2(b), minimum value1/2(b)
  Trans_max_static/1 -> If Action 2/1("Trans_max_static ")
  If1/2 -> If Action 2/Action
  V_eRL/1 -> If1/2
  V_eRR/1 -> If1/1
  If Action 2/1(Trans_limit) -> Merge2/2
  Trans_max_dynamic/1 -> If Action 1/1(Trans_max_dynamic)
  Merge2/1 -> minimum value1/1(a), minimum value/1(a)
  If Action 1/1(Trans_limit) -> Merge2/1
  If1/1 -> If Action 1/Action

== system TV_2021/Vehicle Dynamics Control 1/VDC 2018 without Longitudinal/Constraints/Braking with Regenerative ==
  MaxRegTorque : Inport
  Tq_RR_wc : Inport  Port=2
  Tq_RL_wc : Inport  Port=3
  Action Port : ActionPort
  Gain : Gain  Gain=-1
  Gain1 : Gain  Gain=-1
  MATLAB Function : MATLAB Function  TreatAsAtomicUnit=on
  TQ_RR : Outport
  TQ_RL : Outport  Port=2
  wires:
  Gain/1 -> TQ_RR/1
  Gain1/1 -> TQ_RL/1
  MaxRegTorque/1 -> MATLAB Function/1(MaxRegenTq)
  Tq_RL_wc/1 -> MATLAB Function/3(Tq_RL)
  Tq_RR_wc/1 -> MATLAB Function/2(Tq_RR)
  MATLAB Function/1(RegTq_RR) -> Gain/1
  MATLAB Function/2(RegTq_RL) -> Gain1/1
